simulink model "sak_02"  (R2019b)
settings: Solver=VariableStepAuto  StartTime=0.0  StopTime=10.0  RelTol=1e-3
values from neighbouring files (symbols this model uses):
  s = tf('s')    [kp4_zadach7_Na.m]
libraries: slctrlblks x3
settings Model: Creator=pssaf  LastModifiedBy=pssaf

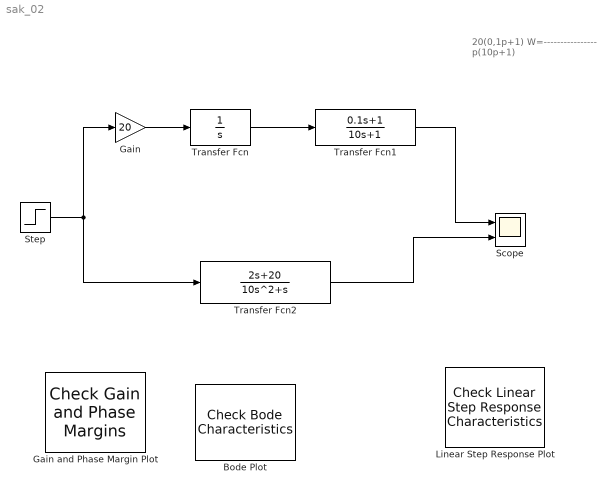
== system sak_02 ==
  note: 20(0,1p+1)
      | W=----------------
      | p(10p+1)
  Bode Plot : slctrlblks/Model Verification/Check Bode  Characteristics  InstantiateOnLoad=on  SaveOperatingPoints=off  LinearizationIOs={'/Step', 1, 'in', 'off', '';'/Transfer Fcn1', 1, 'out', 'off', ''}  LinearizeAt=SnapshotTimes  SnapshotTimes=[0]  TriggerType=rising  SampleTime=auto  RateConversionMethod=zoh  PreWarpFreq=10  UseExactDelayModel=off  UseFullBlockNameLabels=off  UseBusSignalLabels=off  enabled=on  stopWhenAssertionFail=off  export=off  ViewDlgPos=[100 200 510 390]  OpenViewOnLoad=off  LaunchViewOnOpen=off  FrequencyUnits=rad/s  MagnitudeUnits=dB  PhaseUnits=deg  TimeUnits=seconds  EnableUpperBound=off  UpperBoundFrequencies=[]  UpperBoundMagnitudes=[]  EnableLowerBound=off  LowerBoundFrequencies=[]  LowerBoundMagnitudes=[]
      settings: SourceProductName=Simulink Control Design
  Gain : Gain  Gain=20
  Gain and Phase Margin Plot : slctrlblks/Model Verification/Check Gain and Phase Margins  InstantiateOnLoad=on  SaveOperatingPoints=off  LinearizationIOs={'/Step', 1, 'in', 'off', '';'/Transfer Fcn1', 1, 'out', 'off', ''}  LinearizeAt=SnapshotTimes  SnapshotTimes=[0]  TriggerType=rising  SampleTime=auto  RateConversionMethod=zoh  PreWarpFreq=10  UseExactDelayModel=off  UseFullBlockNameLabels=off  UseBusSignalLabels=off  enabled=on  stopWhenAssertionFail=off  export=off  ViewDlgPos=[100 200 510 390]  LaunchViewOnOpen=off  OpenViewOnLoad=off  FrequencyUnits=rad/s  MagnitudeUnits=dB  PhaseUnits=deg  TimeUnits=seconds  EnableMargins=off  GainMargin=[]  PhaseMargin=[]  PlotType=nyquist  FeedbackSign=-1
      settings: SourceProductName=Simulink Control Design  SourceProductBaseCode=SD  SaveToWorkspace=off  SaveName=sys
  Linear Step Response Plot : slctrlblks/Model Verification/Check Linear Step Response Characteristics  InstantiateOnLoad=on  SaveOperatingPoints=off  LinearizationIOs={'/Step', 1, 'in', 'off', '';'/Transfer Fcn1', 1, 'out', 'off', ''}  LinearizeAt=SnapshotTimes  SnapshotTimes=[0]  TriggerType=rising  SampleTime=auto  RateConversionMethod=zoh  PreWarpFreq=10  UseExactDelayModel=off  UseFullBlockNameLabels=off  UseBusSignalLabels=off  enabled=on  stopWhenAssertionFail=off  export=off  ViewDlgPos=[100 200 510 390]  OpenViewOnLoad=off  LaunchViewOnOpen=off  FrequencyUnits=rad/s  MagnitudeUnits=dB  PhaseUnits=deg  TimeUnits=seconds  EnableStepResponseBound=off  FinalValue=[]  RiseTime=[]  PercentRise=[]  SettlingTime=[]  PercentSettling=[]  PercentOvershoot=[]  PercentUndershoot=[]
      settings: SourceProductName=Simulink Control Design  SourceProductBaseCode=SD  SaveToWorkspace=off  SaveName=sys
  Scope : Scope  NumInputPorts=2
  Step : Step  Time=0  SampleTime=0
  Transfer Fcn : TransferFcn  Denominator=[1 0]
  Transfer Fcn1 : TransferFcn  Numerator=[0.1 1]  Denominator=[10 1]
  Transfer Fcn2 : TransferFcn  Numerator=[2 20]  Denominator=[10 1 0]
  wires:
  Gain/1 -> Transfer Fcn/1
  Transfer Fcn/1 -> Transfer Fcn1/1
  Step/1 -> Transfer Fcn2/1, Gain/1
  Transfer Fcn1/1 -> Scope/1
  Transfer Fcn2/1 -> Scope/2
